simulink library "downlink_4c2t_foldingcfr_3firs_lib"  (Simulink 8.7)
settings: Solver=ode45  StartTime=0.0  StopTime=10.0  RelTol=1e-3
undefined symbols (not defined in the file or in its folder): AdvDSPBChannelOutDisplay, Anti, cfr_Params, dpoly, dspba_ChannelInVis, dspba_ChannelOutVis, dspba_internal_get_channel_ports, evalAionMaskParam, Folding, latency, primtype, REG, Symmetrical, value
undefined symbols (not defined in the file): cfr0_id, cfr_angle_cord_bits, cfr_angle_cord_fractional_bits, cfr_stages, cfr_xy_cord_bits, cfr_xy_cord_fractional_bits, clock_rate, DUC_LINEUP_param, REG_dut_id_addr, sample_rate
libraries: DSPBAPrim x74, CORDIC_lib x18, FoldingCFR_3FIRs_lib x16, DSPBAFilters x4, DSPBAModelBus x3, DSPBABase x3
(part 2 of 2)

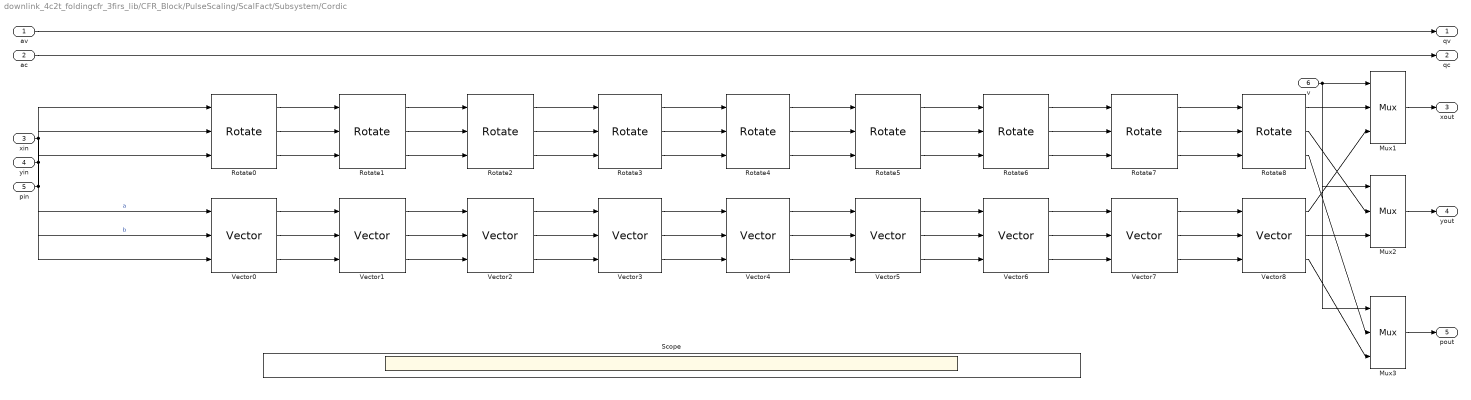
== system downlink_4c2t_foldingcfr_3firs_lib/CFR_Block/PulseScaling/ScalFact/Subsystem/Cordic ==
  av : Inport
  ac : Inport  Port=2
  xin : Inport  Port=3
  yin : Inport  Port=4
  pin : Inport  Port=5
  v : Inport  Port=6
  Mux1 : DSPBAPrim/Mux  primtype=mux  nInputs=evalAionMaskParam(gcb,'value',1)+1  nOutputs=1  omode=Inherit via internal rule  otype=sfix(16)  scale=2^-15  rndmethod=Unbiased  factor=1  satmethod=Symmetric  shift_vec=[0 1 2 -1]  value=2  inPortNames=['s'; 'd0'; 'd1'; 'd2'; 'd3'; 'd4'; 'd5'; 'd6'; 'd7'; 'd8'; 'd9';]  outPortNames=[' ']  dspbaimage=dspba_prim.jpg  text=fprintf('%s', primtype);  style=Optimised  visibilities=1032  version=20131025
  Mux2 : DSPBAPrim/Mux  primtype=mux  nInputs=evalAionMaskParam(gcb,'value',1)+1  nOutputs=1  omode=Inherit via internal rule  otype=sfix(16)  scale=2^-15  rndmethod=Unbiased  factor=1  satmethod=Symmetric  shift_vec=[0 1 2 -1]  value=2  inPortNames=['s'; 'd0'; 'd1'; 'd2'; 'd3'; 'd4'; 'd5'; 'd6'; 'd7'; 'd8'; 'd9';]  outPortNames=[' ']  dspbaimage=dspba_prim.jpg  text=fprintf('%s', primtype);  style=Optimised  visibilities=1032  version=20131025
  Mux3 : DSPBAPrim/Mux  primtype=mux  nInputs=evalAionMaskParam(gcb,'value',1)+1  nOutputs=1  omode=Inherit via internal rule  otype=sfix(16)  scale=2^-15  rndmethod=Unbiased  factor=1  satmethod=Symmetric  shift_vec=[0 1 2 -1]  value=2  inPortNames=['s'; 'd0'; 'd1'; 'd2'; 'd3'; 'd4'; 'd5'; 'd6'; 'd7'; 'd8'; 'd9';]  outPortNames=[' ']  dspbaimage=dspba_prim.jpg  text=fprintf('%s', primtype);  style=Optimised  visibilities=1032  version=20131025
  Rotate0 : CORDIC_lib/Rotate  stage=0  angle_bits=15  angle_frac_bits=15  xy_bits=18  xy_frac_bits=14
  Rotate1 : CORDIC_lib/Rotate  stage=1  angle_bits=15  angle_frac_bits=15  xy_bits=18  xy_frac_bits=14
  Rotate2 : CORDIC_lib/Rotate  stage=2  angle_bits=15  angle_frac_bits=15  xy_bits=18  xy_frac_bits=14
  Rotate3 : CORDIC_lib/Rotate  stage=3  angle_bits=15  angle_frac_bits=15  xy_bits=18  xy_frac_bits=14
  Rotate4 : CORDIC_lib/Rotate  stage=4  angle_bits=15  angle_frac_bits=15  xy_bits=18  xy_frac_bits=14
  Rotate5 : CORDIC_lib/Rotate  stage=5  angle_bits=15  angle_frac_bits=15  xy_bits=18  xy_frac_bits=14
  Rotate6 : CORDIC_lib/Rotate  stage=6  angle_bits=15  angle_frac_bits=15  xy_bits=18  xy_frac_bits=14
  Rotate7 : CORDIC_lib/Rotate  stage=7  angle_bits=15  angle_frac_bits=15  xy_bits=18  xy_frac_bits=14
  Rotate8 : CORDIC_lib/Rotate  stage=8  angle_bits=15  angle_frac_bits=15  xy_bits=18  xy_frac_bits=14
  Scope : Scope  NumInputPorts=9
  Vector0 : CORDIC_lib/Vector  stage=0  angle_bits=15  angle_frac_bits=15  xy_bits=18  xy_frac_bits=14
  Vector1 : CORDIC_lib/Vector  stage=1  angle_bits=15  angle_frac_bits=15  xy_bits=18  xy_frac_bits=14
  Vector2 : CORDIC_lib/Vector  stage=2  angle_bits=15  angle_frac_bits=15  xy_bits=18  xy_frac_bits=14
  Vector3 : CORDIC_lib/Vector  stage=3  angle_bits=15  angle_frac_bits=15  xy_bits=18  xy_frac_bits=14
  Vector4 : CORDIC_lib/Vector  stage=4  angle_bits=15  angle_frac_bits=15  xy_bits=18  xy_frac_bits=14
  Vector5 : CORDIC_lib/Vector  stage=5  angle_bits=15  angle_frac_bits=15  xy_bits=18  xy_frac_bits=14
  Vector6 : CORDIC_lib/Vector  stage=6  angle_bits=15  angle_frac_bits=15  xy_bits=18  xy_frac_bits=14
  Vector7 : CORDIC_lib/Vector  stage=7  angle_bits=15  angle_frac_bits=15  xy_bits=18  xy_frac_bits=14
  Vector8 : CORDIC_lib/Vector  stage=8  angle_bits=15  angle_frac_bits=15  xy_bits=18  xy_frac_bits=14
  qv : Outport
  qc : Outport  Port=2
  xout : Outport  Port=3
  yout : Outport  Port=4
  pout : Outport  Port=5
  wires:
  av/1 -> qv/1
  ac/1 -> qc/1
  xin/1 -> Rotate0/1, Vector0/1  "a"
  yin/1 -> Rotate0/2, Vector0/2  "b"
  pin/1 -> Rotate0/3, Vector0/3
  Rotate0/1 -> Rotate1/1
  Vector0/1 -> Vector1/1
  Rotate0/2 -> Rotate1/2
  Vector0/2 -> Vector1/2
  Rotate0/3 -> Rotate1/3
  Vector0/3 -> Vector1/3
  Rotate1/1 -> Rotate2/1
  Vector1/1 -> Vector2/1
  Rotate1/2 -> Rotate2/2
  Vector1/2 -> Vector2/2
  Rotate1/3 -> Rotate2/3
  Vector1/3 -> Vector2/3
  Rotate2/1 -> Rotate3/1
  Vector2/1 -> Vector3/1
  Rotate2/2 -> Rotate3/2
  Vector2/2 -> Vector3/2
  Rotate2/3 -> Rotate3/3
  Vector2/3 -> Vector3/3
  Rotate3/1 -> Rotate4/1
  Vector3/1 -> Vector4/1
  Rotate3/2 -> Rotate4/2
  Vector3/2 -> Vector4/2
  Rotate3/3 -> Rotate4/3
  Vector3/3 -> Vector4/3
  Rotate4/1 -> Rotate5/1
  Vector4/1 -> Vector5/1
  Rotate4/2 -> Rotate5/2
  Vector4/2 -> Vector5/2
  Rotate4/3 -> Rotate5/3
  Vector4/3 -> Vector5/3
  Rotate5/1 -> Rotate6/1
  Vector5/1 -> Vector6/1
  Rotate5/2 -> Rotate6/2
  Vector5/2 -> Vector6/2
  Rotate5/3 -> Rotate6/3
  Vector5/3 -> Vector6/3
  Rotate6/1 -> Rotate7/1
  Vector6/1 -> Vector7/1
  Rotate6/2 -> Rotate7/2
  Vector6/2 -> Vector7/2
  Rotate6/3 -> Rotate7/3
  Vector6/3 -> Vector7/3
  Rotate7/1 -> Rotate8/1
  Vector7/1 -> Vector8/1
  Rotate7/2 -> Rotate8/2
  Vector7/2 -> Vector8/2
  Rotate7/3 -> Rotate8/3
  Vector7/3 -> Vector8/3
  v/1 -> Mux1/1, Mux2/1, Mux3/1
  Rotate8/1 -> Mux1/2
  Vector8/1 -> Mux1/3
  Rotate8/2 -> Mux2/2
  Vector8/2 -> Mux2/3
  Rotate8/3 -> Mux3/2
  Vector8/3 -> Mux3/3
  Mux1/1 -> xout/1
  Mux2/1 -> yout/1
  Mux3/1 -> pout/1

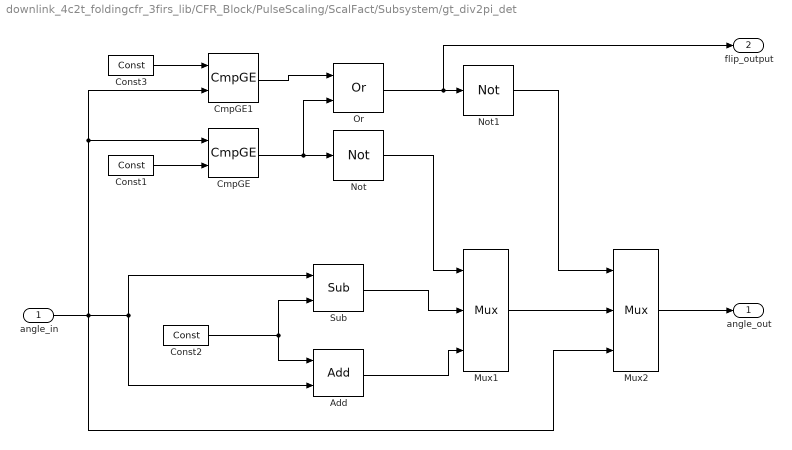
== system downlink_4c2t_foldingcfr_3firs_lib/CFR_Block/PulseScaling/ScalFact/Subsystem/gt_div2pi_det ==
  angle_in : Inport
  Add : DSPBAPrim/Add  primtype=add  nInputs=evalAionMaskParam(gcb,'value',1)  nOutputs=1  omode=Inherit via internal rule with word growth  otype=sfix(16)  scale=2^-15  rndmethod=Unbiased  factor=1  satmethod=Symmetric  shift_vec=[0 1 2 -1]  value=2  inPortNames=[' '; ' ';]  outPortNames=[' ']  dspbaimage=dspba_prim.jpg  text=fprintf('+');  style=Optimised  visibilities=1032  genFPC=off  floatRounding=correct  advOptions=[]  version=20130821
  CmpGE : DSPBAPrim/CmpGE  primtype=cmpgte  nInputs=2  nOutputs=1  omode=boolean  otype=sfix(16)  scale=2^-15  rndmethod=Unbiased  factor=1  satmethod=Symmetric  shift_vec=[0 1 2 -1]  value=0  inPortNames=['a'; 'b';]  outPortNames=[' ']  dspbaimage=dspba_prim.jpg  text=fprintf('a>=b');  style=Optimised  visibilities=0  advOptions=[]  version=20130117
  CmpGE1 : DSPBAPrim/CmpGE  primtype=cmpgte  nInputs=2  nOutputs=1  omode=boolean  otype=sfix(16)  scale=2^-15  rndmethod=Unbiased  factor=1  satmethod=Symmetric  shift_vec=[0 1 2 -1]  value=0  inPortNames=['a'; 'b';]  outPortNames=[' ']  dspbaimage=dspba_prim.jpg  text=fprintf('a>=b');  style=Optimised  visibilities=0  advOptions=[]  version=20130117
  Const1 : DSPBAPrim/Const  primtype=const  nInputs=0  nOutputs=1  omode=Specify via dialog  otype=sfix(angle_bits)  scale=2^-(angle_bits-3)  rndmethod=Unbiased  factor=1  satmethod=Symmetric  shift_vec=[0 1 2 -1]  value=pi/2  inPortNames=['+'; '+';]  outPortNames=[' ']  dspbaimage=dspba_prim.jpg  text=fprintf('%s', num2str(value));  style=Optimised  visibilities=8 + 1024  floatPrecision=float32_m23  version=20120820
  Const2 : DSPBAPrim/Const  primtype=const  nInputs=0  nOutputs=1  omode=Specify via dialog  otype=sfix(angle_bits)  scale=2^-(angle_bits-3)  rndmethod=Unbiased  factor=1  satmethod=Symmetric  shift_vec=[0 1 2 -1]  value=pi/2  inPortNames=['+'; '+';]  outPortNames=[' ']  dspbaimage=dspba_prim.jpg  text=fprintf('%s', num2str(value));  style=Optimised  visibilities=8 + 1024  floatPrecision=float32_m23  version=20120820
  Const3 : DSPBAPrim/Const  primtype=const  nInputs=0  nOutputs=1  omode=Specify via dialog  otype=sfix(angle_bits)  scale=2^-(angle_bits-3)  rndmethod=Unbiased  factor=1  satmethod=Symmetric  shift_vec=[0 1 2 -1]  value=-pi/2  inPortNames=['+'; '+';]  outPortNames=[' ']  dspbaimage=dspba_prim.jpg  text=fprintf('%s', num2str(value));  style=Optimised  visibilities=8 + 1024  floatPrecision=float32_m23  version=20120820
  Mux1 : DSPBAPrim/Mux  primtype=mux  nInputs=evalAionMaskParam(gcb,'value',1)+1  nOutputs=1  omode=Inherit via internal rule  otype=sfix(16)  scale=2^-15  rndmethod=Unbiased  factor=1  satmethod=Symmetric  shift_vec=[0 1 2 -1]  value=2  inPortNames=['s'; 'd0'; 'd1'; 'd2'; 'd3'; 'd4'; 'd5'; 'd6'; 'd7'; 'd8'; 'd9';]  outPortNames=[' ']  dspbaimage=dspba_prim.jpg  text=fprintf('%s', primtype);  style=Optimised  visibilities=1032  version=20131025
  Mux2 : DSPBAPrim/Mux  primtype=mux  nInputs=evalAionMaskParam(gcb,'value',1)+1  nOutputs=1  omode=Inherit via internal rule  otype=sfix(16)  scale=2^-15  rndmethod=Unbiased  factor=1  satmethod=Symmetric  shift_vec=[0 1 2 -1]  value=2  inPortNames=['s'; 'd0'; 'd1'; 'd2'; 'd3'; 'd4'; 'd5'; 'd6'; 'd7'; 'd8'; 'd9';]  outPortNames=[' ']  dspbaimage=dspba_prim.jpg  text=fprintf('%s', primtype);  style=Optimised  visibilities=1032  version=20131025
  Not : DSPBAPrim/Not  primtype=not  nInputs=1  nOutputs=1  omode=Inherit via internal rule  otype=sfix(16)  scale=2^-15  rndmethod=Unbiased  factor=1  satmethod=Symmetric  shift_vec=[0 1 2 -1]  value=0  inPortNames=[' '; ' ';]  outPortNames=[' ']  dspbaimage=dspba_prim.jpg  text=fprintf('~');  style=Optimised  visibilities=8  version=20090407
  Not1 : DSPBAPrim/Not  primtype=not  nInputs=1  nOutputs=1  omode=Inherit via internal rule  otype=sfix(16)  scale=2^-15  rndmethod=Unbiased  factor=1  satmethod=Symmetric  shift_vec=[0 1 2 -1]  value=0  inPortNames=[' '; ' ';]  outPortNames=[' ']  dspbaimage=dspba_prim.jpg  text=fprintf('~');  style=Optimised  visibilities=8  version=20090407
  Or : DSPBAPrim/Or  primtype=or  nInputs=2  nOutputs=1  omode=Inherit via internal rule  otype=sfix(16)  scale=2^-15  rndmethod=Unbiased  factor=1  satmethod=Symmetric  shift_vec=[0 1 2 -1]  value=0  inPortNames=[' '; ' '; ' '; ' '; ' '; ' '; ' '; ' '; ' '; ' '; ' '; ' '; ' '; ' '; ' '; ' '; ]  outPortNames=[' ']  dspbaimage=dspba_prim.jpg  text=fprintf('|');  style=Optimised  visibilities=8+2  version=20090407
  Sub : DSPBAPrim/Sub  primtype=sub  nInputs=2  nOutputs=1  omode=Inherit via internal rule with word growth  otype=sfix(16)  scale=2^-15  rndmethod=Unbiased  factor=1  satmethod=Symmetric  shift_vec=[0 1 2 -1]  value=0  inPortNames=['+'; '-';]  outPortNames=[' ']  dspbaimage=dspba_prim.jpg  text=fprintf('-');  style=Optimised  visibilities=8  floatRounding=correct  advOptions=[]  version=20130115
  angle_out : Outport
  flip_output : Outport  Port=2
  wires:
  Sub/1 -> Mux1/2
  Const2/1 -> Sub/2, Add/1
  Add/1 -> Mux1/3
  angle_in/1 -> Sub/1, Add/2, CmpGE/1, CmpGE1/2, Mux2/3
  Mux2/1 -> angle_out/1
  Const1/1 -> CmpGE/2
  CmpGE/1 -> Not/1, Or/2
  Not/1 -> Mux1/1
  Const3/1 -> CmpGE1/1
  Mux1/1 -> Mux2/2
  Not1/1 -> Mux2/1
  Or/1 -> Not1/1, flip_output/1
  CmpGE1/1 -> Or/1

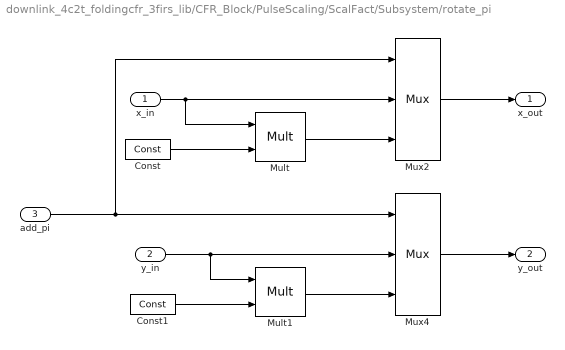
== system downlink_4c2t_foldingcfr_3firs_lib/CFR_Block/PulseScaling/ScalFact/Subsystem/rotate_pi ==
  x_in : Inport
  y_in : Inport  Port=2
  add_pi : Inport  Port=3
  Const : DSPBAPrim/Const  primtype=const  nInputs=0  nOutputs=1  omode=Specify via dialog  otype=sfix(2)  scale=2^-0  rndmethod=Unbiased  factor=1  satmethod=Symmetric  shift_vec=[0 1 2 -1]  value=-1  inPortNames=['+'; '+';]  outPortNames=[' ']  dspbaimage=dspba_prim.jpg  text=fprintf('%s', num2str(value));  style=Optimised  visibilities=8 + 1024  floatPrecision=float32_m23  version=20120820
  Const1 : DSPBAPrim/Const  primtype=const  nInputs=0  nOutputs=1  omode=Specify via dialog  otype=sfix(2)  scale=2^-0  rndmethod=Unbiased  factor=1  satmethod=Symmetric  shift_vec=[0 1 2 -1]  value=-1  inPortNames=['+'; '+';]  outPortNames=[' ']  dspbaimage=dspba_prim.jpg  text=fprintf('%s', num2str(value));  style=Optimised  visibilities=8 + 1024  floatPrecision=float32_m23  version=20120820
  Mult : DSPBAPrim/Mult  primtype=mult  nInputs=2  nOutputs=1  omode=Inherit via internal rule  otype=sfix(16)  scale=2^-15  rndmethod=Unbiased  factor=1  satmethod=Symmetric  shift_vec=[0 1 2 -1]  value=0  inPortNames=[' '; ' ';]  outPortNames=[' ']  dspbaimage=dspba_prim.jpg  text=fprintf('X');  style=Optimised  visibilities=8  floatPrecision=float32_m23  floatRounding=correct  advOptions=[]  version=20130115
  Mult1 : DSPBAPrim/Mult  primtype=mult  nInputs=2  nOutputs=1  omode=Inherit via internal rule  otype=sfix(16)  scale=2^-15  rndmethod=Unbiased  factor=1  satmethod=Symmetric  shift_vec=[0 1 2 -1]  value=0  inPortNames=[' '; ' ';]  outPortNames=[' ']  dspbaimage=dspba_prim.jpg  text=fprintf('X');  style=Optimised  visibilities=8  floatPrecision=float32_m23  floatRounding=correct  advOptions=[]  version=20130115
  Mux2 : DSPBAPrim/Mux  primtype=mux  nInputs=evalAionMaskParam(gcb,'value',1)+1  nOutputs=1  omode=Inherit via internal rule  otype=sfix(16)  scale=2^-15  rndmethod=Unbiased  factor=1  satmethod=Symmetric  shift_vec=[0 1 2 -1]  value=2  inPortNames=['s'; 'd0'; 'd1'; 'd2'; 'd3'; 'd4'; 'd5'; 'd6'; 'd7'; 'd8'; 'd9';]  outPortNames=[' ']  dspbaimage=dspba_prim.jpg  text=fprintf('%s', primtype);  style=Optimised  visibilities=1032  version=20131025
  Mux4 : DSPBAPrim/Mux  primtype=mux  nInputs=evalAionMaskParam(gcb,'value',1)+1  nOutputs=1  omode=Inherit via internal rule  otype=sfix(16)  scale=2^-15  rndmethod=Unbiased  factor=1  satmethod=Symmetric  shift_vec=[0 1 2 -1]  value=2  inPortNames=['s'; 'd0'; 'd1'; 'd2'; 'd3'; 'd4'; 'd5'; 'd6'; 'd7'; 'd8'; 'd9';]  outPortNames=[' ']  dspbaimage=dspba_prim.jpg  text=fprintf('%s', primtype);  style=Optimised  visibilities=1032  version=20131025
  x_out : Outport
  y_out : Outport  Port=2
  wires:
  Mult/1 -> Mux2/3
  Mux4/1 -> y_out/1
  Mux2/1 -> x_out/1
  y_in/1 -> Mux4/2, Mult1/1
  Const1/1 -> Mult1/2
  x_in/1 -> Mux2/2, Mult/1
  Mult1/1 -> Mux4/3
  add_pi/1 -> Mux4/1, Mux2/1
  Const/1 -> Mult/2
